simulink model "SIM2_monophase"  (R2017a)
settings: Solver=VariableStepAuto  StartTime=0.0  StopTime=.2  RelTol=1e-3
values from neighbouring files (symbols this model uses):
  st_time = 10e-3    (= 0.01)    [PR_discretization_2.m]
  st_time3 = 40e-3    (= 0.04)    [PR_discretization_2.m]
libraries: fl_lib x16, nesl_utility x7, elec_lib x3, powerlib_meascontrol x1
settings Model: Creator=erich  LastModifiedBy=erich

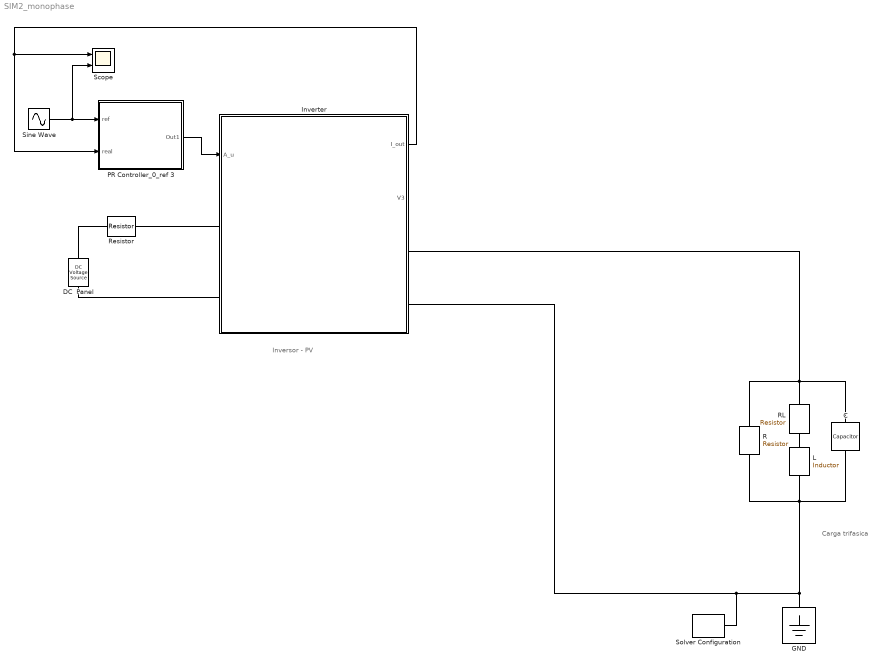
== system SIM2_monophase ==
  note: Carga trifasica
  note: Inversor - PV
  C : fl_lib/Electrical/Electrical Elements/Capacitor  c=100e-6 uF  r=1e-6 Ohm  g=0 1/Ohm  i_specify=off  i_priority=None  i=0 A  i_nominal_specify=off  i_nominal_unit=A  i_nominal_value=1  v_specify=off  v_priority=None  v=0 V  v_nominal_specify=off  v_nominal_unit=V  v_nominal_value=1  vc_specify=off  vc_priority=High  vc=0 V  vc_nominal_specify=off  vc_nominal_unit=V  vc_nominal_value=1
  DC  Panel : elec_lib/Additional Components/SPICE-Compatible Components/Sources/DC Voltage Source  DC=340 V
      settings: SourceProductName=Simscape Electronics  SourceProductBaseCode=SN
  GND : fl_lib/Electrical/Electrical Elements/Electrical Reference
  Inverter : Subsystem
      mask Display:
      | port_label('input', 1, 'Mos IN')
      | 
      | port_label('lconn', 1, 'DC +')
      | port_label('lconn', 2, 'DC -')
      | 
      | 
      | port_label('rconn', 1, 'out +')
      | port_label('rconn', 2, 'out -')
      | 
      | 
      | port_label('output', 1, 'I_out', 'texmode', 'on')
      | port_label('output', 2, 'V_out', 'texmode', 'on')
      | 
      | plot([0.1 .9], [0.1 .9])
      | plot([0.2 .4], [.7 .7])
      | plot([0.2 .24], [.65 .65])
      | plot([0.28 .32], [.65 .65])
      | plot([0.36 .40], [.65 .65])
      | 
      | plot([.5:.01:.7], .25+sin(30*[.2:.01:.4])/10)
  L : fl_lib/Electrical/Electrical Elements/Inductor  l=5200 mH  r=0 Ohm  g=100e-9 1/Ohm  i_specify=off  i_priority=None  i=0 A  i_nominal_specify=off  i_nominal_unit=A  i_nominal_value=1  v_specify=off  v_priority=None  v=0 V  v_nominal_specify=off  v_nominal_unit=V  v_nominal_value=1  i_L_specify=off  i_L_priority=High  i_L=0 A  i_L_nominal_specify=off  i_L_nominal_unit=A  i_L_nominal_value=1
  PR Controller_0_ref 3 : Subsystem
      mask Display:
      | port_label('input',1,'ref')
      | port_label('input',2,'sens')
      | port_label('output',1,'out')
  R : fl_lib/Electrical/Electrical Elements/Resistor  R=15 Ohm  i_specify=off  i_priority=None  i=0 A  i_nominal_specify=off  i_nominal_unit=A  i_nominal_value=1  v_specify=off  v_priority=None  v=0 V  v_nominal_specify=off  v_nominal_unit=V  v_nominal_value=1
  RL : elec_lib/Passive Devices/Resistor  R=1 Ohm  R_tol=5  enable_R_tol=0  tol_distribution=1  nSigma=4  enable_operating_limits=0  operating_limit_action=2  max_working_voltage=100 V  power_rating=1 W  enable_faults=0  fault_action=1  R_faulted=inf Ohm  enable_temporal_fault=0  t_fault=1 s  enable_behavioral_fault=0  max_permissible_current=1 A  t_fail_on_current=1 s  noise_mode=0  sample_time=1e-3 s  repeatability=1  auto_seed=1234795251  user_seed=0  Tdevice=25 degC  alpha=3.93e-3 1/K  Tmeas=25 degC  thermal_mass=100 J/K  power_derating_T1=70 degC  power_derating_T2=155 degC  operating_temperature_range_vec=[-50.0, 150.0] degC  temperature_specify=off  temperature_priority=High  temperature=298.15 K  temperature_nominal_specify=off  temperature_nominal_unit=K  temperature_nominal_value=1
  Resistor : elec_lib/Passive Devices/Resistor  R=.1 Ohm  R_tol=5  enable_R_tol=0  tol_distribution=1  nSigma=4  enable_operating_limits=0  operating_limit_action=2  max_working_voltage=100 V  power_rating=1 W  enable_faults=0  fault_action=1  R_faulted=inf Ohm  enable_temporal_fault=0  t_fault=1 s  enable_behavioral_fault=0  max_permissible_current=1 A  t_fail_on_current=1 s  noise_mode=0  sample_time=1e-3 s  repeatability=1  auto_seed=1274213173  user_seed=0  Tdevice=25 degC  alpha=3.93e-3 1/K  Tmeas=25 degC  thermal_mass=100 J/K  power_derating_T1=70 degC  power_derating_T2=155 degC  operating_temperature_range_vec=[-50.0, 150.0] degC  temperature_specify=off  temperature_priority=High  temperature=298.15 K  temperature_nominal_specify=off  temperature_nominal_unit=K  temperature_nominal_value=1
  Scope : Scope  NumInputPorts=2
  Sine Wave : Sin  Amplitude=20  Frequency=2*pi*60  SampleTime=0
  Solver Configuration : nesl_utility/Solver Configuration  PhysicalDomain=network_engine_domain  SubClassName=solver  LeftPortType=input  RightPortType=generic  Accelerate=off  Tones=[]  Harmonics=[]  SimulateNoise=off  Profile=off  UseLocalSampling=off  EnableSwitchedLinearOptims=on  FrequencyDomain=off  UseCCode=off  RelTol=0.001  AbsTol=1e-06  MinStep=1e-09  ToWorkspace=off  RevertToSquareIcSolve=off  NumHomotopyIterations=100  PhasorMode=off  PhasorModeNumHarmonics=1  OverrideAbsTol=off  DoDC=off  ResidualTolerance=1e-09  UseLocalSolver=on  LocalSolverChoice=NE_BACKWARD_EULER_ADVANCER  LocalSolverSampleTime=1e-6  DoFixedCost=on  MaxNonlinIter=3  MaxModeIter=2  LinearAlgebra=Sparse  DelaysMemoryBudget=1024  AutomaticFiltering=on  FilteringTimeConstant=0.001
  wires:
  PR Controller_0_ref 3/1(Out1) -> Inverter/1(A_u)
  Sine Wave/1 -> Scope/2, PR Controller_0_ref 3/1(ref)
  Inverter/1(I_out) -> PR Controller_0_ref 3/2(real), Scope/1
  connections:
  Resistor/LConn1 -- DC  Panel/LConn1
  DC  Panel/RConn1 -- Inverter/LConn2
  Resistor/RConn1 -- Inverter/LConn1
  C/LConn1 -- RL/LConn1 -- R/LConn1 -- Inverter/RConn1
  Solver Configuration/RConn1 -- C/RConn1 -- L/RConn1 -- R/RConn1 -- GND/LConn1 -- Inverter/RConn2
  RL/RConn1 -- L/LConn1

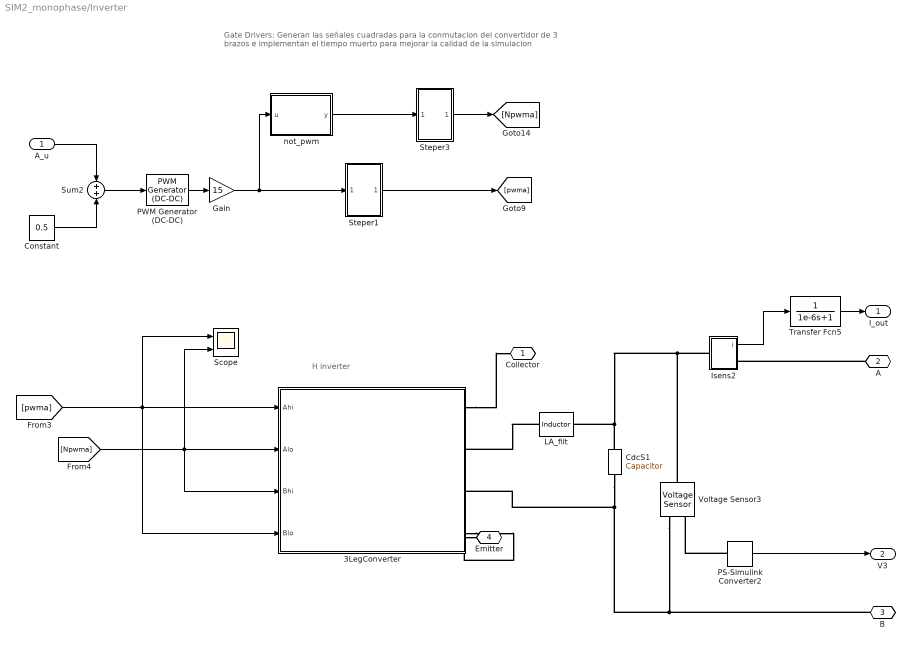
== system SIM2_monophase/Inverter ==
  note: Gate Drivers: Generan las señales cuadradas para
      | la conmutacion del convertidor de 3 brazos e implementan el
      | tiempo muerto para mejorar la calidad de la simulacion
  note: H inverter
  A_u : Inport
  3LegConverter : Subsystem
      mask Display:
      | % entradas de conmutacion del mosfet
      | port_label('input',1,'Ahi')
      | port_label('input',2,'Alo')
      | port_label('input',3,'Bhi')
      | port_label('input',4,'Blo')
      | 
      | 
      | % puertos de conexion del inversor
      | port_label('rconn',1,'Collector') % + fuente dc
      | port_label('rconn',2,'Out +') % fase A
      | port_label('rconn',3,'Out -') % fase B
      | port_label('rconn',4,'Emitter') % ref fuente dc
      | 
      | 
      | plot([.4 .4],[.35 .7])
      | plot([.2 .4],[.52 .52])
      | plot([.46 .46],[.22 .85])
      | plot([.46 .7],[.73 .73])
      | plot([.46 .7],[.32 .32])
  CdcS1 : fl_lib/Electrical/Electrical Elements/Capacitor  c=3.5 uF  r=1e-6 Ohm  g=0 1/Ohm  i_specify=off  i_priority=None  i=0 A  i_nominal_specify=off  i_nominal_unit=A  i_nominal_value=1  v_specify=off  v_priority=None  v=0 V  v_nominal_specify=off  v_nominal_unit=V  v_nominal_value=1  vc_specify=on  vc_priority=High  vc=0 V  vc_nominal_specify=off  vc_nominal_unit=V  vc_nominal_value=1
  Constant : Constant  Value=0.5
  Gain : Gain  Gain=15
  Isens2 : Subsystem
  LA_filt : fl_lib/Electrical/Electrical Elements/Inductor  l=6.2 mH  r=0.1 Ohm  g=1e-6 1/Ohm  i_specify=off  i_priority=None  i=0 A  i_nominal_specify=off  i_nominal_unit=A  i_nominal_value=1  v_specify=off  v_priority=None  v=0 V  v_nominal_specify=off  v_nominal_unit=V  v_nominal_value=1  i_L_specify=on  i_L_priority=High  i_L=0 A  i_L_nominal_specify=off  i_L_nominal_unit=A  i_L_nominal_value=1
  PS-Simulink Converter2 : nesl_utility/PS-Simulink Converter  PhysicalDomain=network_engine_domain  SubClassName=ps_output  LeftPortType=input  RightPortType=output  PseudoPeriodic=off  Frequencies=[]  Unit=1  AffineConversion=off
  PWM Generator (DC-DC) : powerlib_meascontrol/Pulse & Signal Generators/PWM Generator (DC-DC)  Fsw=5000  Ts=0
  Scope : Scope  NumInputPorts=2
  Steper1 : Subsystem
  Steper3 : Subsystem
  Sum2 : Sum
  Transfer Fcn5 : TransferFcn  Denominator=[1e-6 1]
  Voltage Sensor3 : fl_lib/Electrical/Electrical Sensors/Voltage Sensor
  not_pwm : MATLAB Function  TreatAsAtomicUnit=on
  Collector : PMIOPort  Port=1  Side=Left
  A : PMIOPort  Port=2  Side=Right
  B : PMIOPort  Port=3  Side=Right
  Emitter : PMIOPort  Port=4  Side=Left
  I_out : Outport
  V3 : Outport  Port=2
  wires:
  [pwma] -> 3LegConverter/4(Blo), Scope/1, 3LegConverter/1(Ahi)
  [Npwma] -> 3LegConverter/3(Bhi), Scope/2, 3LegConverter/2(Alo)
  Gain/1 -> Steper1/1(In1), not_pwm/1(u)
  Steper3/1(Out1) -> [Npwma]
  Constant/1 -> Sum2/2
  Sum2/1 -> PWM Generator (DC-DC)/1
  not_pwm/1(y) -> Steper3/1(In1)
  PWM Generator (DC-DC)/1 -> Gain/1
  Steper1/1(Out1) -> [pwma]
  A_u/1 -> Sum2/1
  Isens2/1(i) -> Transfer Fcn5/1
  PS-Simulink Converter2/1 -> V3/1
  Transfer Fcn5/1 -> I_out/1
  connections:
  3LegConverter/RConn4 -- Emitter/RConn1
  3LegConverter/RConn1 -- Collector/RConn1
  A/RConn1 -- Isens2/RConn1
  PS-Simulink Converter2/LConn1 -- Voltage Sensor3/RConn1
  CdcS1/RConn1 -- Isens2/LConn1 -- Voltage Sensor3/LConn1 -- LA_filt/RConn1
  LA_filt/LConn1 -- 3LegConverter/RConn2
  CdcS1/LConn1 -- B/RConn1 -- Voltage Sensor3/RConn2 -- 3LegConverter/RConn3

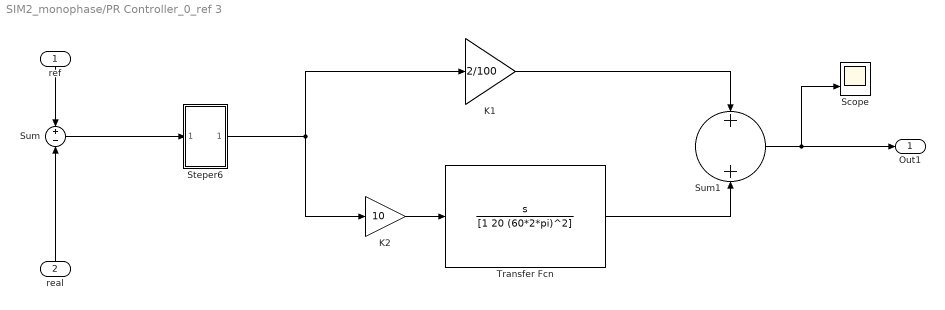
== system SIM2_monophase/PR Controller_0_ref 3 ==
  ref : Inport
  real : Inport  Port=2
  K1 : Gain  Gain=2/100
  K2 : Gain  Gain=10
  Scope : Scope  NumInputPorts=2
  Steper6 : Subsystem
  Sum : Sum  Inputs=+-
  Sum1 : Sum  Inputs=+|+
  Transfer Fcn : TransferFcn  Numerator=[1 0]  Denominator=[1 20 (60*2*pi)^2]
  Out1 : Outport
  wires:
  real/1 -> Sum/2
  ref/1 -> Sum/1
  Sum/1 -> Steper6/1(In1)
  K1/1 -> Sum1/1
  Transfer Fcn/1 -> Sum1/2
  K2/1 -> Transfer Fcn/1
  Steper6/1(Out1) -> K1/1, K2/1
  Sum1/1 -> Scope/2, Out1/1

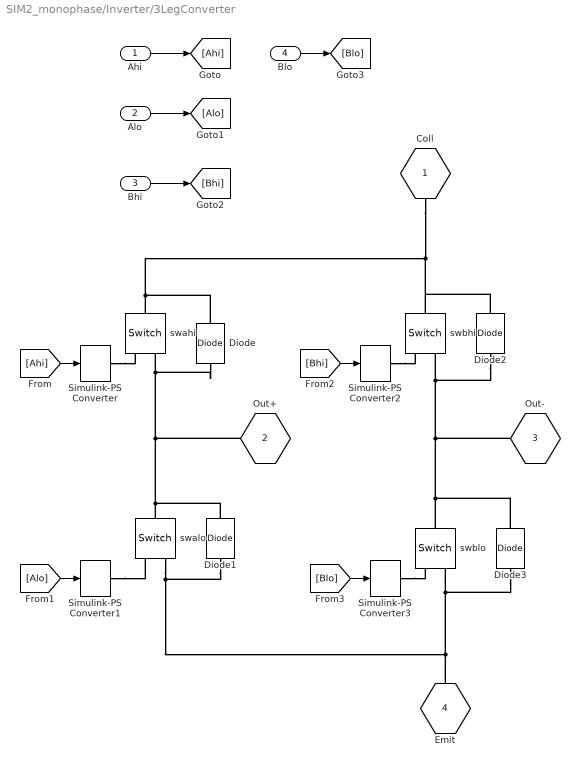
== system SIM2_monophase/Inverter/3LegConverter ==
  Ahi : Inport
  Alo : Inport  Port=2
  Bhi : Inport  Port=3
  Blo : Inport  Port=4
  Diode{,1..3} (4 alike) : fl_lib/Electrical/Electrical Elements/Diode  Vf=0.6 V  Ron=0.3 Ohm  Goff=1e-8 1/Ohm  i_specify=off  i_priority=None  i=0 A  i_nominal_specify=off  i_nominal_unit=A  i_nominal_value=1  v_specify=off  v_priority=None  v=0 V  v_nominal_specify=off  v_nominal_unit=V  v_nominal_value=1
  Simulink-PS Converter{,1..3} (4 alike) : nesl_utility/Simulink-PS Converter  PhysicalDomain=network_engine_domain  SubClassName=ps_input  LeftPortType=input  RightPortType=output  PseudoPeriodic=off  Frequencies=[]  NoiseDistribution=none  NoiseParameters=[]  Unit=1  AffineConversion=off  FilteringAndDerivatives=zero  SimscapeFilterOrder=1  InputFilterTimeConstant=0.001  UdotUserProvided=1
  swahi : fl_lib/Electrical/Electrical Elements/Switch  R_closed=0.01 Ohm  G_open=1e-8 1/Ohm  Threshold=2  i_specify=off  i_priority=None  i=0 A  i_nominal_specify=off  i_nominal_unit=A  i_nominal_value=1  v_specify=off  v_priority=None  v=0 V  v_nominal_specify=off  v_nominal_unit=V  v_nominal_value=1
      settings: SourceProductName=Simscape
  swalo : fl_lib/Electrical/Electrical Elements/Switch  R_closed=0.01 Ohm  G_open=1e-8 1/Ohm  Threshold=2  i_specify=off  i_priority=None  i=0 A  i_nominal_specify=off  i_nominal_unit=A  i_nominal_value=1  v_specify=off  v_priority=None  v=0 V  v_nominal_specify=off  v_nominal_unit=V  v_nominal_value=1
      settings: SourceProductName=Simscape
  swbhi : fl_lib/Electrical/Electrical Elements/Switch  R_closed=0.01 Ohm  G_open=1e-8 1/Ohm  Threshold=2  i_specify=off  i_priority=None  i=0 A  i_nominal_specify=off  i_nominal_unit=A  i_nominal_value=1  v_specify=off  v_priority=None  v=0 V  v_nominal_specify=off  v_nominal_unit=V  v_nominal_value=1
      settings: SourceProductName=Simscape
  swblo : fl_lib/Electrical/Electrical Elements/Switch  R_closed=0.01 Ohm  G_open=1e-8 1/Ohm  Threshold=2  i_specify=off  i_priority=None  i=0 A  i_nominal_specify=off  i_nominal_unit=A  i_nominal_value=1  v_specify=off  v_priority=None  v=0 V  v_nominal_specify=off  v_nominal_unit=V  v_nominal_value=1
      settings: SourceProductName=Simscape
  Coll : PMIOPort  Port=1  Side=Right
  Out+ : PMIOPort  Port=2  Side=Right
  Out- : PMIOPort  Port=3  Side=Right
  Emit : PMIOPort  Port=4  Side=Right
  wires:
  [Alo] -> Simulink-PS Converter1/1
  [Ahi] -> Simulink-PS Converter/1
  Alo/1 -> [Alo]
  [Blo] -> Simulink-PS Converter3/1
  Bhi/1 -> [Bhi]
  [Bhi] -> Simulink-PS Converter2/1
  Ahi/1 -> [Ahi]
  Blo/1 -> [Blo]
  connections:
  swalo/RConn2 -- Diode3/LConn1 -- swblo/RConn2 -- Emit/RConn1 -- Diode1/LConn1
  Simulink-PS Converter/RConn1 -- swahi/RConn1
  swblo/LConn1 -- Diode3/RConn1 -- Out-/RConn1 -- Diode2/LConn1 -- swbhi/RConn2
  Simulink-PS Converter3/RConn1 -- swblo/RConn1
  Simulink-PS Converter2/RConn1 -- swbhi/RConn1
  Simulink-PS Converter1/RConn1 -- swalo/RConn1
  swalo/LConn1 -- Out+/RConn1 -- Diode/LConn1 -- swahi/RConn2 -- Diode1/RConn1
  swahi/LConn1 -- Diode/RConn1 -- Coll/RConn1 -- Diode2/RConn1 -- swbhi/LConn1

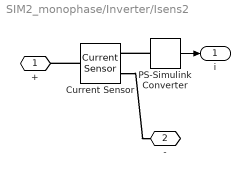
== system SIM2_monophase/Inverter/Isens2 ==
  Current Sensor : fl_lib/Electrical/Electrical Sensors/Current Sensor
  PS-Simulink Converter : nesl_utility/PS-Simulink Converter  PhysicalDomain=network_engine_domain  SubClassName=ps_output  LeftPortType=input  RightPortType=output  PseudoPeriodic=off  Frequencies=[]  Unit=1  AffineConversion=off
  + : PMIOPort  Port=1  Side=Left
  - : PMIOPort  Port=2  Side=Right
  i : Outport
  wires:
  PS-Simulink Converter/1 -> i/1
  connections:
  PS-Simulink Converter/LConn1 -- Current Sensor/RConn1
  Current Sensor/RConn2 -- -/RConn1
  Current Sensor/LConn1 -- +/RConn1

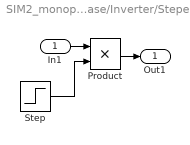
== system SIM2_monophase/Inverter/Steper1 ==
  In1 : Inport
  Product : Product
  Step : Step  Time=st_time3  SampleTime=0
  Out1 : Outport
  wires:
  Step/1 -> Product/2
  In1/1 -> Product/1
  Product/1 -> Out1/1

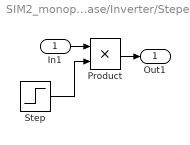
== system SIM2_monophase/Inverter/Steper3 ==
  In1 : Inport
  Product : Product
  Step : Step  Time=st_time3  SampleTime=0
  Out1 : Outport
  wires:
  Product/1 -> Out1/1
  In1/1 -> Product/1
  Step/1 -> Product/2

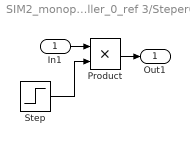
== system SIM2_monophase/PR Controller_0_ref 3/Steper6 ==
  In1 : Inport
  Product : Product
  Step : Step  Time=st_time  SampleTime=0
  Out1 : Outport
  wires:
  Product/1 -> Out1/1
  In1/1 -> Product/1
  Step/1 -> Product/2

== matlab function SIM2_monophase/Inverter/not_pwm ==
  data: u input; y output
function y = fcn(u)
%#codegen

if(u==0 || u<0)
    a=15;
else
    a=0;
end;

y = a;
